simulink model "Serial_Subsystem"  (R2022a)
settings: Solver=FixedStepAuto  StartTime=0.0  StopTime=10.0  FixedStep=1e-3  RelTol=1e-3  EnableMultiTasking=on
libraries: frdmk64flib x1
settings Model: ExtModeTrigDuration=5  Creator=bmile  LastModifiedBy=bmile
settings OptimizationCC: EnhancedBackFolding=on  PassReuseOutputArgsAs=Individual arguments  ZeroExternalMemoryAtStartup=off  ZeroInternalMemoryAtStartup=off  MaxStackSize=64  OptimizeBlockOrder=speed  DifferentSizesBufferReuse=on  OptimizationCustomize=off  EfficientTunableParamExpr=on
settings DebuggingCC: ParameterTunabilityLossMsg=error
settings HardwareCC: ProdBitPerPointer=32  ProdBitPerSizeT=32  ProdBitPerPtrDiffT=32  ProdLargestAtomicInteger=Long  ProdLargestAtomicFloat=Double  ProdWordSize=32  ProdHWDeviceType=ARM Compatible->ARM Cortex
settings SFSimCC: MATLABDynamicMemAlloc=off
settings RTWCC: SystemTargetFile=ert.tlc  HardwareBoard=NXP FRDM-K64F  TLCOptions="-aInlineSetEventsForThisBaseRateFcn=TLC_FALSE -aSuppressMultiTaskScheduler=TLC_FALSE  -aRateBasedStepFcn=0"  TemplateMakefile=ert_default_tmf  Toolchain=GNU Tools for ARM Embedded Processors
settings CodeAppCC: ForceParamTrailComments=on  IgnoreCustomStorageClasses=off  OperatorAnnotations=on  SimulinkDataObjDesc=on  SFDataObjDesc=on  InsertBlockDesc=on
settings ERTTargetCC: ExtModeTransport=4  ExtModeMexFile=sendToCommService

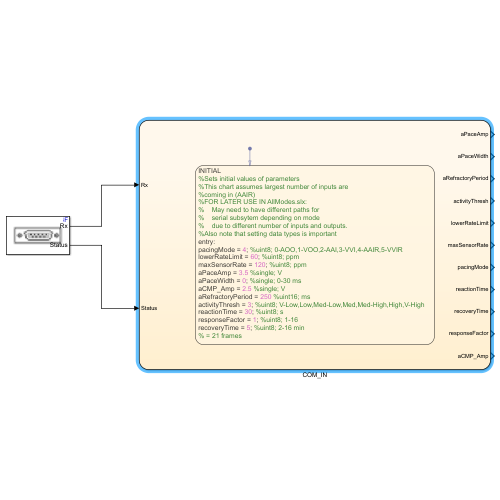
[thumbnail: Simulink's stored preview of the top-level diagram]
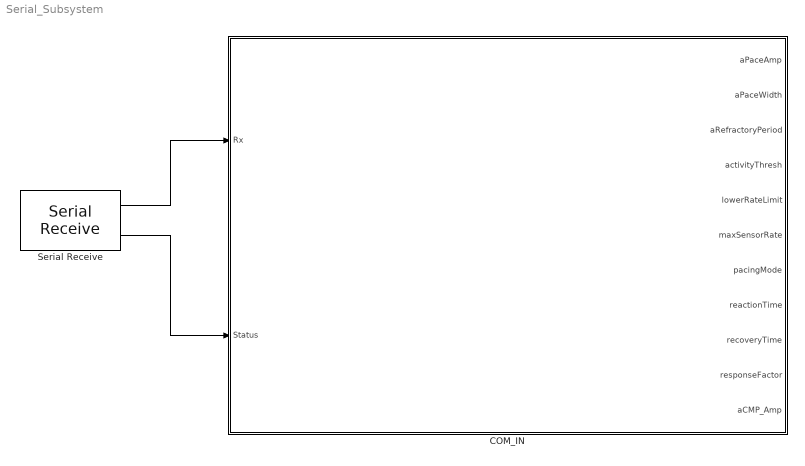
== system Serial_Subsystem ==
  COM_IN : Stateflow chart  TreatAsAtomicUnit=on
  Serial Receive : frdmk64flib/Serial Receive  SCIModule=0  Baudrate=uint32(9600)  Parity=None  StopBits=1  HardwareFlowControl=None  ByteOrder=LittleEndian  DataType=uint8  DataLength=10  BlockingMode=off  OutputStatus=on  SampleTime=0.1
  wires:
  Serial Receive/1 -> COM_IN/1(Rx)
  Serial Receive/2 -> COM_IN/2(Status)

== stateflow chart Serial_Subsystem/COM_IN ==
  state INITIAL
    %Sets initial values of parameters
    %This chart assumes largest number of inputs are
    %coming in (AAIR)
    %FOR LATER USE IN AllModes.slx:
    %    May need to have different paths for
    %    serial subsytem depending on mode
    %    due to different number of inputs and outputs.
    %Also note that setting data types is important
    entry:
    pacingMode = 4; %uint8; 0-AOO,1-VOO,2-AAI,3-VVI,4-AAIR,5-VVIR
    lowerRateLimit = 60; %uint8; ppm
    maxSensorRate = 120; %uint8; ppm
    aPaceAmp = 3.5 %single; V
    aPaceWidth = 0; %single; 0-30 ms
    aCMP_Amp = 2.5 %single; V
    aRefractoryPeriod = 250 %uint16; ms
    activityThresh = 3; %uint8; V-Low,Low,Med-Low,Med,Med-High,High,V-High
    reactionTime = 30; %uint8; s
    responseFactor = 1; %uint8; 1-16
    recoveryTime = 5; %uint8; 2-16 min
    % = 21 frames
  (default) -> INITIAL
  data: Rx input; Status input; aPaceAmp output single; aPaceWidth output single; aRefractoryPeriod output uint16; activityThresh output uint8; lowerRateLimit output uint8; maxSensorRate output uint8; pacingMode output uint8; reactionTime output uint8; recoveryTime output uint8; responseFactor output uint8; aCMP_Amp output single
